simulink model "dummy_beamformer"  (Simulink 9.2)
settings: Solver=VariableStepDiscrete  StartTime=0.0  StopTime=dummy_beamformer_param.endTime  RelTol=1e-3  EnableMultiTasking=on
PreLoadFcn:
  | % Run the setup script when the model is opened
  | setup_dummy_beamformer;
InitFcn:
  | % Run the setup script again just before the
  | % model is run, so that any updates made
  | % after opening are applied.
  | setup_dummy_beamformer;
undefined symbols (not defined in the file or in its folder): AdvDSPBChannelOutDisplay, dspba_ChannelInVis, dspba_ChannelOutVis, dspba_internal_get_channel_ports, dspba_internal_get_demux_ports, dummy_beamformer_param, evalAionMaskParam, latency, value
libraries: DSPBAPrim x10, DSPBABase x3, simulink x3, dpsba_custom x2
Description:
  | DSP Builder Advanced Template for Template Design implementing ModelIP designs
settings Model: LogicAnalyzerSignalOrdering=d749b274-2e9b-41f7-821b-efb3867ad4af,9dbc4500-4deb-4713-b377-808ae297f30c,1cf25e40-dad1-4891-9461-5262ed41fef7,3d876275-4dcb-4596-ba7a-8aabfee40974,dba767da-77d0-46e0-bf7a-e2725d6c63da,e6e660a1-e70d-4a7f-8863-c003ac4afc31,e894caa8-2371-4756-9ac3-514711069f4e,99b00191-1232-48c7-b334-08b1405adb5d,f756ead7-aa7e-4cad-ad20-6b4cd5dd4375,5905b608-676e-40a2-a514-7330fa9507ae,2019b513-c153-4e29-9cd7-289924617150,4c808de4-5e6b-4dde-ab15-06a681e2f2f2,8fcfe0ac-d5cb-4cd4-8fb9-04297cb389b6,4e624832-9380-46d7-ab66-16e5181ae136,34d06037-172e-40ba-9423-b8bcb513c834,e55b9da5-5cab-4880-8590-92b7e1dc1cef,f1ba8934-d78a-4446-a73c-f718dfc8a558,a061eb46-72e7-4a44-a63e-37f0d008ee0a,923ed878-3fa4-4f1d-9a8a-34518576e425,f8c57ebb-1970-4521-a661-f02f35922478,83740012-9601-4ea8-a6be-8846b47f3600,5f1c7f20-f126-4b33-8246-199eb0a90ef3,69cac0b3-e8e4-4c89-befa-051451c0a906,3db69d68-307d-4d4a-95e2-0fe81ab176ba,1265ac64-3139-4adc-9244-2dc0b3386e0e,540753a4-b171-4194-83df-3567500bc965,de3e0426-42d3-42a2-b072-560502f54d48,110e8d3f-44ac-46b9-9cdc-f0a090d178dd  Creator=mjervis  LastModifiedBy=trevorvannoy
settings Model: LogicAnalyzerGraphicalSettings=|
  | {
  |   "cursors" : {
  |     "activeCursor" : 0,
  |     "lockedCursors" : [
  | 
  |     ],
  |     "startingCursor" : 0,
  |     "times" : [
  |       3275
  |     ]
  |   },
  |   "global" : {
  |     "backgroundColor" : "#ffffff",
  |     "booleanDisplay" : "gradient",
  |     "color" : "#0073bd",
  |     "displayBusElementNames" : true,
  |     "displayShortNames" : true,
  |     "recentlyUsedColors" : [
  |       "default",
  |       "#ffff11",
  |       "#139fff",
  |       "#ff6929",
  |       "#64d413",
  |       "#b746ff",
  |       "#0fffff"
  |     ]
  |   },
  |   "panels" : [
  |     {
  |       "height" : 100,
  |       "startingTrace" : 8,
  |       "traces" : [
  |         {
  |           "color" : "#d9541a",
  |           "fontSize" : 16,
  |           "height" : 24,
  |           "signalId" : "9dbc4500-4deb-4713-b377-808ae297f30c",
  |           "type" : "wave"
  |         },
  |         {
  |           "color" : "#d9541a",
  |           "fontSize" : 16,
  |           "height" : 24,
  |           "signalId" : "d749b274-2e9b-41f7-821b-efb3867ad4af",
  |           "type" : "wave"
  |         },
  |         {
  |           "color" : "#d9541a",
  |           "fontSize" : 16,
  |           "height" : 24,
  |           "radix" : "signeddecimal",
  |           "signalId" : "1cf25e40-dad1-4891-9461-5262ed41fef7",
  |           "type" : "wave"
  |         },
  |         {
  |           "color" : "#0073bd",
  |           "fontSize" : 16,
  |           "height" : 24,
  |           "radix" : "signeddecimal",
  |           "signalId" : "3d876275-4dcb-4596-ba7a-8aabfee40974",
  |           "type" : "wave"
  |         },
  |         {
  |           "color" : "#0073bd",
  |           "fontSize" : 16,
  |           "height" : 24,
  |           "radix" : "signeddecimal",
  |           "signalId" : "dba767da-77d0-46e0-bf7a-e2725d6c63da",
  |           "type" : "wave"
  |         },
  |         {
  |           "color" : "#0073bd",
  |           "fontSize" : 16,
  |           "height" : 24,
  |           "radix" : "signeddecimal",
  |           "signalId" : "e6e660a1-e70d-4a7f-8863-c003ac4afc31",
  |           "type" : "wave"
  |         },
  |         {
  |           "color" : "#0073bd",
  |           "fontSize" : 16,
  |           "height" : 24,
  |           "radix" : "signeddecimal",
  |           "signalId" : "e894caa8-2371-4756-9ac3-514711069f4e",
  |           "type" : "wave"
  |         },
  |         {
  |           "color" : "#0073bd",
  |           "fontSize" : 16,
  |           "height" : 24,
  |           "radix" : "signeddecimal",
  |           "signalId" : "99b00191-1232-48c7-b334-08b1405adb5d",
  |           "type" : "wave"
  |         },
  |         {
  |           "color" : "#0073bd",
  |           "fontSize" : 16,
  |           "height" : 24,
  |           "radix" : "signeddecimal",
  |           "signalId" : "f756ead7-aa7e-4cad-ad20-6b4cd5dd4375",
  |           "type" : "wave"
  |         },
  |         {
  |           "color" : "#0073bd",
  |           "fontSize" : 16,
  |           "height" : 24,
  |           "radix" : "signeddecimal",
  |           "signalId" : "5905b608-676e-40a2-a514-7330fa9507ae",
  |           "type" : "wave"
  |         },
  |         {
  |           "color" : "#0073bd",
  |           "fontSize" : 16,
  |           "height" : 24,
  |           "radix" : "signeddecimal",
  |           "signalId" : "4c808de4-5e6b-4dde-ab15-06a681e2f2f2",
  |           "type" : "wave"
  |         },
  |         {
  |           "color" : "#0073bd",
  |           "fontSize" : 16,
  |           "height" : 24,
  |           "radix" : "signeddecimal",
  |           "signalId" : "8fcfe0ac-d5cb-4cd4-8fb9-04297cb389b6",
  |           "type" : "wave"
  |         },
  |         {
  |           "color" : "#0073bd",
  |           "fontSize" : 16,
  |           "height" : 24,
  |           "radix" : "signeddecimal",
  |           "signalId" : "4e624832-9380-46d7-ab66-16e5181ae136",
  |           "type" : "wave"
  |         },
  |         {
  |           "color" : "#0073bd",
  |           "fontSize" : 16,
  |           "height" : 24,
  |           "radix" : "signeddecimal",
  |           "signalId" : "2019b513-c153-4e29-9cd7-289924617150",
  |           "type" : "wave"
  |         },
  |         {
  |           "color" : "#0073bd",
  |           "fontSize" : 16,
  |           "height" : 24,
  |           "radix" : "signeddecimal",
  |           "signalId" : "34d06037-172e-40ba-9423-b8bcb513c834",
  |           "type" : "wave"
  |         },
  |         {
  |           "color" : "#0073bd",
  |           "fontSize" : 16,
  |           "height" : 24,
  |           "radix" : "signeddecimal",
  |           "signalId" : "e55b9da5-5cab-4880-8590-92b7e1dc1cef",
  |           "type" : "wave"
  |         },
  |         {
  |           "color" : "#0073bd",
  |           "fontSize" : 16,
  |           "height" : 24,
  |           "radix" : "signeddecimal",
  |           "signalId" : "f1ba8934-d78a-4446-a73c-f718dfc8a558",
  |           "type" : "wave"
  |         },
  |         {
  |           "color" : "#0073bd",
  |           "fontSize" : 16,
  |           "height" : 24,
  |           "radix" : "signeddecimal",
  |           "signalId" : "a061eb46-72e7-4a44-a63e-37f0d008ee0a",
  |           "type" : "wave"
  |         },
  |         {
  |           "color" : "#0073bd",
  |           "fontSize" : 16,
  |           "height" : 24,
  |           "radix" : "signeddecimal",
  |           "signalId" : "923ed878-3fa4-4f1d-9a8a-34518576e425",
  |           "type" : "wave"
  |         },
  |         {
  |           "color" : "#edb021",
  |           "fontSize" : 16,
  |           "height" : 24,
  |           "name" : "vout",
  |           "signalId" : "f8c57ebb-1970-4521-a661-f02f35922478",
  |           "type" : "wave"
  |         },
  |         {
  |           "color" : "#edb021",
  |           "fontSize" : 16,
  |           "height" : 24,
  |           "name" : "cout",
  |           "signalId" : "83740012-9601-4ea8-a6be-8846b47f3600",
  |           "type" : "wave"
  |         },
  |         {
  |           "color" : "#edb021",
  |           "fontSize" : 16,
  |           "height" : 24,
  |           "name" : "dout",
  |           "radix" : "signeddecimal",
  |           "signalId" : "5f1c7f20-f126-4b33-8246-199eb0a90ef3",
  |           "type" : "wave"
  |         },
  |         {
  |           "signalId" : "69cac0b3-e8e4-4c89-befa-051451c0a906",
  |           "type" : "wave"
  |         },
  |         {
  |           "signalId" : "3db69d68-307d-4d4a-95e2-0fe81ab176ba",
  |           "type" : "wave"
  |         },
  |         {
  |           "signalId" : "1265ac64-3139-4adc-9244-2dc0b3386e0e",
  |           "type" : "wave"
  |         },
  |         {
  |           "signalId" : "540753a4-b171-4194-83df-3567500bc965",
  |           "type" : "wave"
  |         },
  |         {
  |           "signalId" : "de3e0426-42d3-42a2-b072-560502f54d48",
  |           "type" : "wave"
  |         },
  |         {
  |           "signalId" : "110e8d3f-44ac-46b9-9cdc-f0a090d178dd",
  |           "type" : "wave"
  |         }
  |       ],
  |       "yOffset" : 14
  |     }
  |   ],
  |   "timeAxis" : {
  |     "pixelsPerSecond" : 0.1758
  |   },
  |   "trigger" : {
  |     "enabled" : false,
  |     "mode" : "once",
  |     "samples" : 200,
  |     "signals" : {
  |     },
  |     "stages" : [
  |       {
  |         "conditions" : [
  | 
  |         ],
  |         "operator" : "AND"
  |       }
  |     ]
  |   }
  | }
settings DataIOCC: SignalLoggingSaveFormat=Dataset
settings OptimizationCC: ExpressionDepthLimit=2147483647
settings DebuggingCC: SolverPrmCheckMsg=warning  InheritedTsInSrcMsg=none  IntegerOverflowMsg=none  IntegerSaturationMsg=none

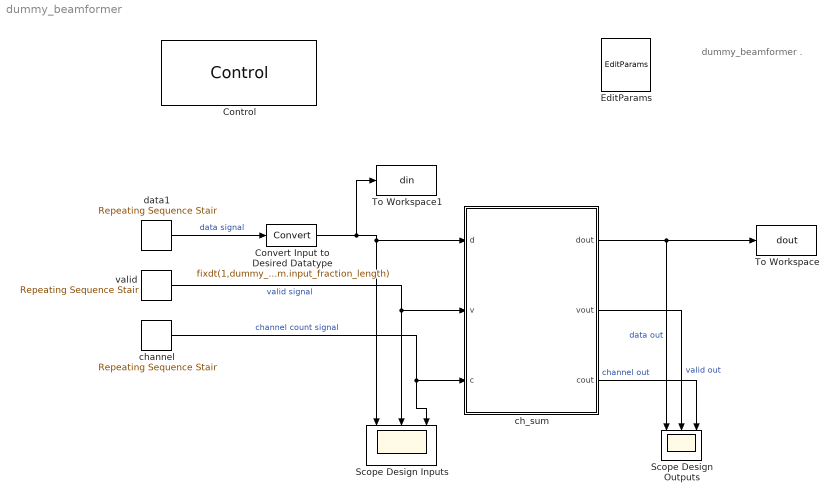
== system dummy_beamformer ==
  note: dummy_beamformer
      |                                          .
  Control : DSPBABase/Control  generate=on  language=VHDL  destination=./rtl  destination_gui=./rtl  make_full_path=off  quartus_work=../rtl  quartus_work_gui=../rtl  path_is_relative=on  autotestbench=on  signaldepth=2  coveragetestbench=off  logs=off  spacewidth=2  spacenum=1  addrwidth=10  datawidth=16  dataendian=Big Endian  hierarchicalnames=off  ramThresholdBits=-1  distRamThresholdBits=-1  mlabThresholdBits=-1  hardMultiplierThresholdLuts=-1  version=20090407  errorOnChanMismatch=on  errorOnGPIOMismatch=off  importModelsimResults=0  floatMismatchTolerance=-1.0  floatMismatchZeroTolerance=-1.0  cycleAccurate=off  reinterpretCastMult=off  paramFile=dummy_beamformer_params.xml
  Convert Input to Desired Datatype : DataTypeConversion  OutDataTypeStr=fixdt(1,dummy_beamformer_param.input_word_length,dummy_beamformer_param.input_fraction_length)  SaturateOnIntegerOverflow=on
  EditParams : DSPBABase/EditParams  version=20090407
  Scope Design Inputs : Scope  NumInputPorts=3
  Scope Design Outputs : Scope  NumInputPorts=3
  To Workspace : ToWorkspace  VariableName=dout  SampleTime=-1
      settings: Save2DSignal=2-D array (concatenate along first dimension)
  To Workspace1 : ToWorkspace  VariableName=din  SampleTime=-1
      settings: Save2DSignal=2-D array (concatenate along first dimension)
  ch_sum : Subsystem
  channel : simulink/Sources/Repeating Sequence Stair  OutValues=dummy_beamformer_param.chan_stim  tsamp=dummy_beamformer_param.ClockCycle  OutMin=[]  OutMax=[]  OutDataTypeStr=uint8  OutputDataTypeScalingMode=uint8  OutDataType=unit8  ConRadixGroup=Best Precision: Vector-wise  OutScaling=[]
  data1 : simulink/Sources/Repeating Sequence Stair  OutValues=dummy_beamformer_param.input_data  tsamp=dummy_beamformer_param.ClockCycle  OutMin=[]  OutMax=[]  OutDataTypeStr=Inherit: Inherit via back propagation  OutDataType=fixdt('sfix16_En15')  ConRadixGroup=Best Precision: Vector-wise  OutScaling=[]
  valid : simulink/Sources/Repeating Sequence Stair  OutValues=[1, zeros(1, dummy_beamformer_param.SampleTime-1)]  tsamp=dummy_beamformer_param.ClockCycle  OutMin=[]  OutMax=[]  OutDataTypeStr=Inherit: Inherit via back propagation  OutDataType=fixdt(0,1,0)  ConRadixGroup=Best Precision: Vector-wise  OutScaling=[]
  wires:
  ch_sum/2(vout) -> Scope Design Outputs/2  "valid out"
  ch_sum/3(cout) -> Scope Design Outputs/3  "channel out"
  ch_sum/1(dout) -> To Workspace/1, Scope Design Outputs/1  "data out"
  valid/1 -> ch_sum/2(v), Scope Design Inputs/2  "valid signal"
  channel/1 -> ch_sum/3(c), Scope Design Inputs/3  "channel count signal"
  Convert Input to Desired Datatype/1 -> To Workspace1/1, ch_sum/1(d), Scope Design Inputs/1
  data1/1 -> Convert Input to Desired Datatype/1  "data signal"

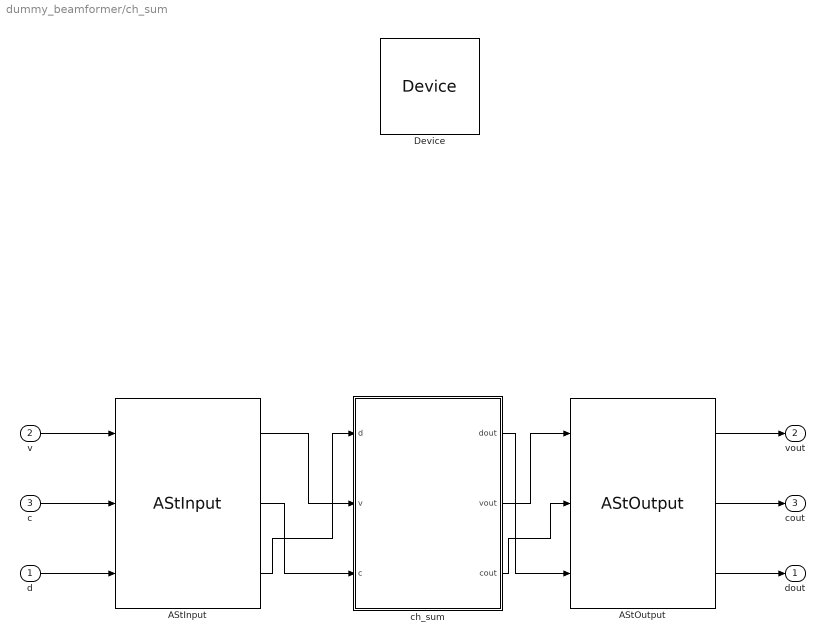
== system dummy_beamformer/ch_sum ==
  d : Inport
  v : Inport  Port=2
  c : Inport  Port=3
  AStInput : dpsba_custom/AStInput
      link override ChannelOut: latency=0
      settings: SourceProductName=Custom DSP Builder Advanced blocks
  AStOutput : dpsba_custom/AStOutput  fifo_setup=[32 1 20]
      link override ChannelOut: latency=0
      settings: SourceProductName=Custom DSP Builder Advanced blocks
  Device : DSPBABase/Device  family=Stratix IV  deviceMember=Stratix IV GX  stratix4device=Stratix IV GX  hardcopy4device=HardCopy IV E  stratix5device=Stratix V GX  device=AUTO  speed=-2  stratixSpeed=-5  stratix2Speed=-3  stratix3Speed=-3  stratix4gxSpeed=-2  stratix4gtSpeed=-1  cyclone2Speed=-6  cyclone3Speed=-7  arria2Speed=-4  cyclone4eSpeed=-8  stratix5Speed=-3  arria5Speed=-4  arriaSpeed=-6  cyclone3lsSpeed=-7  cyclone5Speed=-6  arria2gzSpeed=-3  nightFurySpeed=-2  ecp2Speed=-7  hardcopycompat=off  version=20140217  max10flashmode=off  max10nomeminit=off
  ch_sum : Subsystem
  dout : Outport
  vout : Outport  Port=2
  cout : Outport  Port=3
  wires:
  AStInput/1 -> ch_sum/2(v)
  AStInput/2 -> ch_sum/3(c)
  AStInput/3 -> ch_sum/1(d)
  ch_sum/2(vout) -> AStOutput/1
  ch_sum/1(dout) -> AStOutput/3
  ch_sum/3(cout) -> AStOutput/2
  AStOutput/1 -> vout/1
  AStOutput/2 -> cout/1
  AStOutput/3 -> dout/1
  d/1 -> AStInput/3
  c/1 -> AStInput/2
  v/1 -> AStInput/1

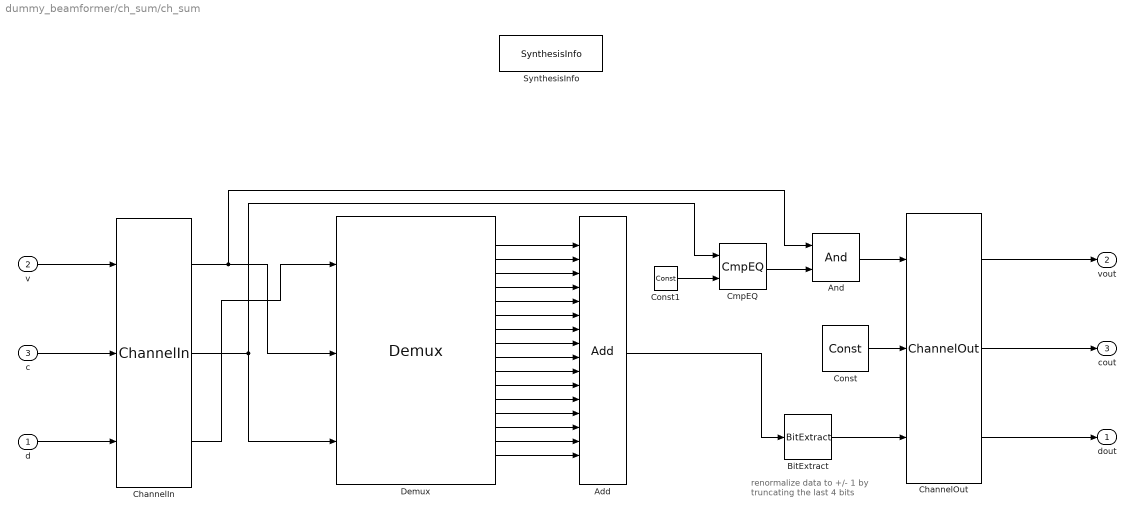
== system dummy_beamformer/ch_sum/ch_sum ==
  note: renormalize data to +/- 1 by truncating the last 4 bits
  d : Inport
  v : Inport  Port=2
  c : Inport  Port=3
  Add : DSPBAPrim/Add  primtype=add  nInputs=evalAionMaskParam(gcb,'value',1)  nOutputs=1  omode=Inherit via internal rule with word growth  otype=sfix(dummy_beamformer_param.output_word_length)  scale=2^(-dummy_beamformer_param.output_fraction_length)  rndmethod=Unbiased  factor=1  satmethod=Symmetric  shift_vec=[0 1 2 -1]  value=16  inPortNames=[' '; ' ';]  outPortNames=[' ']  dspbaimage=dspba_prim.jpg  text=fprintf('+');  style=Optimised  visibilities=1032+2^17+2^18+2^19  genFPC=off  floatRounding=correct  advOptions=[]  version=20130821
  And : DSPBAPrim/And  primtype=and  nInputs=2  nOutputs=1  omode=Inherit via internal rule  otype=sfix(16)  scale=2^-15  rndmethod=Unbiased  factor=1  satmethod=Symmetric  shift_vec=[0 1 2 -1]  value=0  inPortNames=[' '; ' '; ' '; ' '; ' '; ' '; ' '; ' '; ' '; ' '; ' '; ' '; ' '; ' '; ' '; ' '; ]  outPortNames=[' ']  dspbaimage=dspba_prim.jpg  text=fprintf('&');  style=Optimised  visibilities=8+2  version=20090407
  BitExtract : DSPBAPrim/BitExtract  primtype=bitextract  nInputs=1  nOutputs=1  omode=Specify via dialog  otype=sfix(dummy_beamformer_param.output_word_length)  scale=2^(-dummy_beamformer_param.output_fraction_length)  rndmethod=Unbiased  factor=1  satmethod=Symmetric  shift_vec=[0 1 2 -1]  value=4  inPortNames=[' '; ' ';]  outPortNames=[' ']  dspbaimage=dspba_prim.jpg  text=fprintf('..%d', value);  style=Optimised  visibilities=8+1024  version=20090407
  ChannelIn : DSPBAPrim/ChannelIn  primtype=channelin  nInputs=dspba_internal_get_channel_ports(gcb)  nOutputs=dspba_internal_get_channel_ports(gcb)  omode=Inherit via internal rule  otype=sfix(16)  scale=2^-15  rndmethod=Unbiased  factor=1  satmethod=Symmetric  shift_vec=[0 1 2 -1]  value=1  inPortNames=['v'; 'c'; '0'; '1'; '2'; '3'; '4'; '5'; '6'; '7'; '8'; '9'; 'A'; 'B'; 'D'; 'E'; 'F'; 'G'; 'H'; 'I'; 'J'; 'K'; 'L'; 'M'; 'N'; 'O'; 'P'; 'Q'; 'R'; 'S'; 'T'; 'U'; 'W'; 'X'; 'Y'; 'Z']  outPortNames=['v'; 'c'; '0'; '1'; '2'; '3'; '4'; '5'; '6'; '7'; '8'; '9'; 'A'; 'B'; 'D'; 'E'; 'F'; 'G'; 'H'; 'I'; 'J'; 'K'; 'L'; 'M'; 'N'; 'O'; 'P'; 'Q'; 'R'; 'S'; 'T'; 'U'; 'W'; 'X'; 'Y'; 'Z']  dspbaimage=dspba_prim.jpg  text=fprintf('In');  style=Optimised  dataSignals=1  foldingEnabled=off  channels=1  sampleRate=200  packetBeginPresent=off  packetBeginEnabled=off  visibilities=dspba_ChannelInVis(gcb)  latencyCorrection=0  scheduleOrigin=on  version=20141013
  ChannelOut : DSPBAPrim/ChannelOut  primtype=channelout  nInputs=dspba_internal_get_channel_ports(gcb)  nOutputs=dspba_internal_get_channel_ports(gcb)  omode=Inherit via internal rule  otype=sfix(16)  scale=2^-15  rndmethod=Unbiased  factor=1  satmethod=Symmetric  shift_vec=[0 1 2 -1]  value=1  inPortNames=['v'; 'c'; '0'; '1'; '2'; '3'; '4'; '5'; '6'; '7'; '8'; '9'; 'A'; 'B'; 'D'; 'E'; 'F'; 'G'; 'H'; 'I'; 'J'; 'K'; 'L'; 'M'; 'N'; 'O'; 'P'; 'Q'; 'R'; 'S'; 'T'; 'U'; 'W'; 'X'; 'Y'; 'Z']  outPortNames=['v'; 'c'; '0'; '1'; '2'; '3'; '4'; '5'; '6'; '7'; '8'; '9'; 'A'; 'B'; 'D'; 'E'; 'F'; 'G'; 'H'; 'I'; 'J'; 'K'; 'L'; 'M'; 'N'; 'O'; 'P'; 'Q'; 'R'; 'S'; 'T'; 'U'; 'W'; 'X'; 'Y'; 'Z']  dspbaimage=dspba_prim.jpg  text=fprintf('Out%s', AdvDSPBChannelOutDisplay(latency));  style=Optimised  dataSignals=1  foldingEnabled=off  channels=1  sampleRate=200  packetBeginPresent=off  packetBeginEnabled=off  visibilities=dspba_ChannelOutVis(gcb)  latency=2  latencyCorrection=0  version=20141013
  CmpEQ : DSPBAPrim/CmpEQ  primtype=cmpeq  nInputs=2  nOutputs=1  omode=boolean  otype=sfix(16)  scale=2^-15  rndmethod=Unbiased  factor=1  satmethod=Symmetric  shift_vec=[0 1 2 -1]  value=0  inPortNames=[' '; ' ';]  outPortNames=[' ']  dspbaimage=dspba_prim.jpg  text=fprintf('==');  style=Optimised  visibilities=0  advOptions=[]  version=20130117
  Const : DSPBAPrim/Const  primtype=const  nInputs=0  nOutputs=1  omode=Inherit via back propagation  otype=sfix(16)  scale=2^-15  rndmethod=Unbiased  factor=1  satmethod=Symmetric  shift_vec=[0 1 2 -1]  value=0  inPortNames=['+'; '+';]  outPortNames=[' ']  dspbaimage=dspba_prim.jpg  text=fprintf('%s', num2str(value));  style=Optimised  visibilities=8 + 1024  floatPrecision=float32_m23  version=20120820
  Const1 : DSPBAPrim/Const  primtype=const  nInputs=0  nOutputs=1  omode=Inherit via internal rule  otype=sfix(16)  scale=2^-15  rndmethod=Unbiased  factor=1  satmethod=Symmetric  shift_vec=[0 1 2 -1]  value=dummy_beamformer_param.ChanCount-1  inPortNames=['+'; '+';]  outPortNames=[' ']  dspbaimage=dspba_prim.jpg  text=fprintf('%s', num2str(value));  style=Optimised  visibilities=8 + 1024  floatPrecision=float32_m23  version=20120820
  Demux : DSPBAPrim/Demux  primtype=demux  nInputs=3  nOutputs=dspba_internal_get_demux_ports(gcb)  omode=Inherit via internal rule  otype=sfix(16)  scale=2^-15  rndmethod=Unbiased  factor=1  satmethod=Symmetric  shift_vec=[0:dummy_beamformer_param.ChanCount-1]  value=dummy_beamformer_param.ChanCount  inPortNames=['q'; 'v'; 'c']  outPortNames=['c0'; 'c1']  dspbaimage=dspba_prim.jpg  text=fprintf('demux');  style=Optimised  visibilities=1536  version=20100120
  SynthesisInfo : DSPBAPrim/SynthesisInfo  primtype=synthinfo  nInputs=0  nOutputs=0  omode=Inherit via internal rule  otype=sfix(16)  scale=2^-15  rndmethod=Truncate  factor=1  satmethod=Symmetric  shift_vec=[0 1 2 -1]  value=99  inPortNames=[' '; ' ';]  outPortNames=[' ']  dspbaimage=dspba_prim_ctrl.jpg  text=fprintf('Style=%s', style);  style=Scheduled  visibilities=2^17+2^18+2^19+2^20  constraintInUse=off  constraintRelation=>  constraintLimit=2  bitAccurate=off  version=20150220
  dout : Outport
  vout : Outport  Port=2
  cout : Outport  Port=3
  wires:
  Demux/6 -> Add/6
  Demux/4 -> Add/4
  Demux/9 -> Add/9
  ChannelIn/2 -> CmpEQ/1, Demux/3
  Demux/15 -> Add/15
  Demux/11 -> Add/11
  Demux/16 -> Add/16
  Demux/13 -> Add/13
  Demux/5 -> Add/5
  Add/1 -> BitExtract/1
  Const/1 -> ChannelOut/2
  Demux/7 -> Add/7
  Demux/1 -> Add/1
  Const1/1 -> CmpEQ/2
  Demux/12 -> Add/12
  ChannelOut/2 -> cout/1
  ChannelOut/3 -> dout/1
  Demux/3 -> Add/3
  Demux/8 -> Add/8
  d/1 -> ChannelIn/3
  Demux/10 -> Add/10
  Demux/2 -> Add/2
  ChannelIn/3 -> Demux/1
  ChannelOut/1 -> vout/1
  c/1 -> ChannelIn/2
  Demux/14 -> Add/14
  v/1 -> ChannelIn/1
  CmpEQ/1 -> And/2
  And/1 -> ChannelOut/1
  ChannelIn/1 -> And/1, Demux/2
  BitExtract/1 -> ChannelOut/3
